simulink model "CruiseControl_IntCalc"  (R2015b)
settings: Solver=FixedStepDiscrete  StartTime=0.0  StopTime=16  FixedStep=0.1  RelTol=1e-3
PreLoadFcn:
  | CruiseControl_DivByZero_dd;
model workspace (MAT data in the model file):
  min_speed = 20
  min_throttle = 0.6
values from neighbouring files (symbols this model uses):
  holdrate = mpt.Parameter    [CruiseControl_DivByZero_dd.m]
  incdec = mpt.Parameter    [CruiseControl_DivByZero_dd.m]
  maxtspeed = mpt.Parameter    [CruiseControl_DivByZero_dd.m]
  mintspeed = mpt.Parameter    [CruiseControl_DivByZero_dd.m]
libraries: DEDlib x1
settings Model: Creator=The MathWorks Inc.  LastModifiedBy=colosky
settings DataIOCC: SaveFormat=Array  SaveOutput=off  SaveTime=off
settings OptimizationCC: DefaultParameterBehavior=Inlined  InlineInvariantSignals=on  ExpressionDepthLimit=2147483647  InitFltsAndDblsToZero=on
settings DebuggingCC: SaveWithParameterizedLinksMsg=none  UnderspecifiedInitializationDetection=Classic  MergeDetectMultiDrivingBlocksExec=none  SolverPrmCheckMsg=warning  FcnCallInpInsideContextMsg=UseLocalSettings  StateNameClashWarn=warning  StrictBusMsg=ErrorOnBusTreatedAsVector
settings HardwareCC: ProdBitPerPointer=32  ProdLargestAtomicFloat=None  ProdIntDivRoundTo=Undefined  ProdEndianess=Unspecified  ProdWordSize=32  ProdHWDeviceType=32-bit Generic
settings SFSimCC: SimParseCustomCode=off
settings GRTTargetCC: TargetFcnLib=ansi_tfl_tmw.mat  GeneratePreprocessorConditionals=Disable all  CombineOutputUpdateFcns=off  GRTInterface=on
settings ConfigComp: RecordCoverage=on  CovMetricSettings=dcme  CovHtmlReporting=off  CovSaveCumulativeToWorkspaceVar=off  CovSaveSingleToWorkspaceVar=off  CovModelRefEnable=Off  CovSFcnEnable=off  DVMode=DesignErrorDetection  DVMaxProcessTime=3000  DVDisplayUnsatisfiableObjectives=on  DVAutomaticStubbing=off  DVMakeOutputFilesUnique=off  DVParametersConfigFileName=C:\matlab_user\Temp\MAC_MASTER\VnV_MASTER_MAC\Models\DesignErrDetect\CruiseControl_SLDV_ParTable.m  DVModelCoverageObjectives=MCDC  DVMaxTestCaseSteps=500  DVTestSuiteOptimization=CombinedObjectives  DVAssertions=EnableAll  DVProofAssumptions=EnableAll  DVDetectIntegerOverflow=off  DVDetectDeadLogic=on  DVDetectActiveLogic=on  DVMaxViolationSteps=50  DVModelReferenceHarness=on  DVReportIncludeGraphics=on

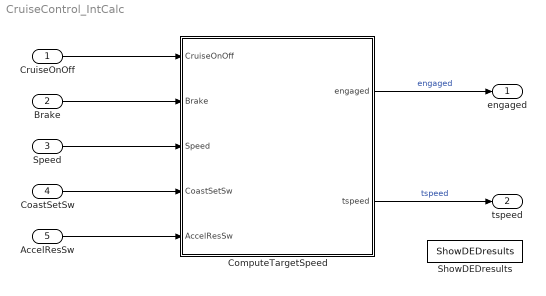
== system CruiseControl_IntCalc ==
  CruiseOnOff : Inport  OutDataTypeStr=boolean  PortDimensions=1
  Brake : Inport  Port=2  OutDataTypeStr=boolean  PortDimensions=1
  Speed : Inport  Port=3  OutDataTypeStr=single  PortDimensions=1
  CoastSetSw : Inport  Port=4  OutDataTypeStr=boolean  PortDimensions=1
  AccelResSw : Inport  Port=5  OutDataTypeStr=boolean  PortDimensions=1
  ComputeTargetSpeed : Stateflow chart  TreatAsAtomicUnit=on
  ShowDEDresults : DEDlib/ShowDEDresults  SystemSampleTime=-1
  engaged : Outport
  tspeed : Outport  Port=2
  wires:
  ComputeTargetSpeed/2(tspeed) -> tspeed/1  "tspeed"
  ComputeTargetSpeed/1(engaged) -> engaged/1  "engaged"
  AccelResSw/1 -> ComputeTargetSpeed/5(AccelResSw)
  CruiseOnOff/1 -> ComputeTargetSpeed/1(CruiseOnOff)
  Brake/1 -> ComputeTargetSpeed/2(Brake)
  CoastSetSw/1 -> ComputeTargetSpeed/4(CoastSetSw)
  Speed/1 -> ComputeTargetSpeed/3(Speed)

== stateflow chart CruiseControl_IntCalc/ComputeTargetSpeed ==
  state OFF
    en:
    engaged = false;
    tspeed = 0;
  state CRUISE
    state ON
      en: engaged = true;
      state Accel
        tspeed = tspeed + incdec;
      state Steady
      state Coast
        tspeed = tspeed - incdec;
      (junction 60) -> Accel
      (junction 57) -> (junction 60) : [after(incdec/holdrate...
          | *uint8(10),tick)]
      Accel -> (junction 57) [order 2]
      Steady -> Accel [order 1] : [hasChangedTo(AccelResSw,true) ...
          | && tspeed < maxtspeed]
      Accel -> Steady [order 1] : [!AccelResSw || ...
          | tspeed > maxtspeed]
      Steady -> (junction 75) [order 3] : [hasChangedTo(CoastSetSw,true)]
      (default) -> (junction 75)
      (junction 75) -> (junction 77) : {tspeed = Speed;}
      (junction 77) -> Steady
      Steady -> Coast [order 2] : [hasChangedTo(CoastSetSw,true) ...
          | && tspeed > mintspeed]
      Coast -> Steady [order 1] : [!CoastSetSw || ...
          | tspeed < mintspeed]
      (junction 72) -> Coast
      (junction 71) -> (junction 72) : [after(incdec/holdrate...
          | *uint8(10),tick)]
      Coast -> (junction 71) [order 2]
    state STANDBY
      en:
      engaged=false;
    (default) -> STANDBY
    ON -> STANDBY : [Brake||Speed> maxtspeed||Speed<mintspeed]
    STANDBY -> (junction 103) : [~Brake && ...
        | Speed<=maxtspeed && ...
        | Speed>=mintspeed]
    (junction 103) -> Steady [order 1] : [hasChangedTo(AccelResSw,true)...
        | &&tspeed!=0]
    (junction 103) -> (junction 106) [order 2]
    (junction 106) -> ON : [hasChangedTo(CoastSetSw,true)]
  (default) -> OFF
  OFF -> CRUISE : [CruiseOnOff]
  CRUISE -> OFF : [~CruiseOnOff]
  data: engaged output boolean; CruiseOnOff input; Brake input; Speed input; CoastSetSw input; AccelResSw input; tspeed output single; incdec parameter; holdrate parameter; maxtspeed parameter; mintspeed parameter
